simulink model "StabilityControllerPosition"  (R2022b)
settings: configuration reference "WheelSimConfiguration2016" (kept outside this file)
undefined symbols (not defined in the file): simulator
settings Model: Creator=At  LastModifiedBy=ateay
settings ConfigSetRef: SourceName=WheelSimConfiguration2016  SourceLocation=Base Workspace

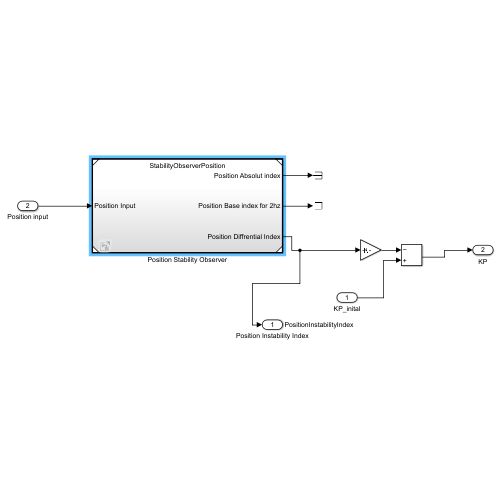
[thumbnail: Simulink's stored preview of the top-level diagram]
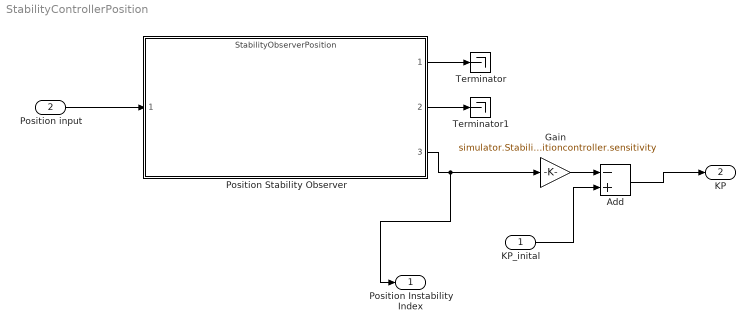
== system StabilityControllerPosition ==
  KP_inital : Inport
  "Position input " : Inport  Port=2
  Add : Sum  Inputs=-+
  Gain : Gain  Gain=simulator.Stabilitypositioncontroller.sensitivity
  Position Stability Observer : ModelReference  ModelNameDialog=StabilityObserverPosition.slx  SimulationMode=Normal  ModelReferenceVersion=1.19
  Terminator : Terminator
  Terminator1 : Terminator
  Position Instability Index : Outport  SignalName=PositionInstabilityIndex
  KP : Outport  Port=2
  wires:
  "Position input "/1 -> Position Stability Observer/1
  Position Stability Observer/1 -> Terminator/1
  Position Stability Observer/2 -> Terminator1/1
  KP_inital/1 -> Add/2
  Gain/1 -> Add/1
  Add/1 -> KP/1
  Position Stability Observer/3 -> Position Instability Index/1, Gain/1
